simulink subsystem "leds"  (R2023b)
settings: Solver=VariableStepAuto  StartTime=0.0  StopTime=10.0  RelTol=1e-3
libraries: simulink x4, arduinolib x3
settings Model: Creator=Usuario_UMA  LastModifiedBy=fdcdm

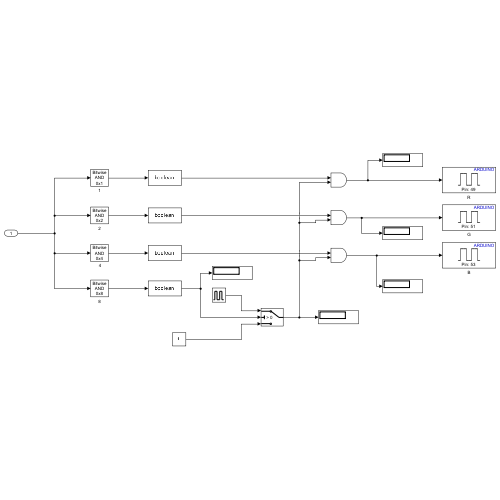
[thumbnail: Simulink's stored preview of the top-level diagram]
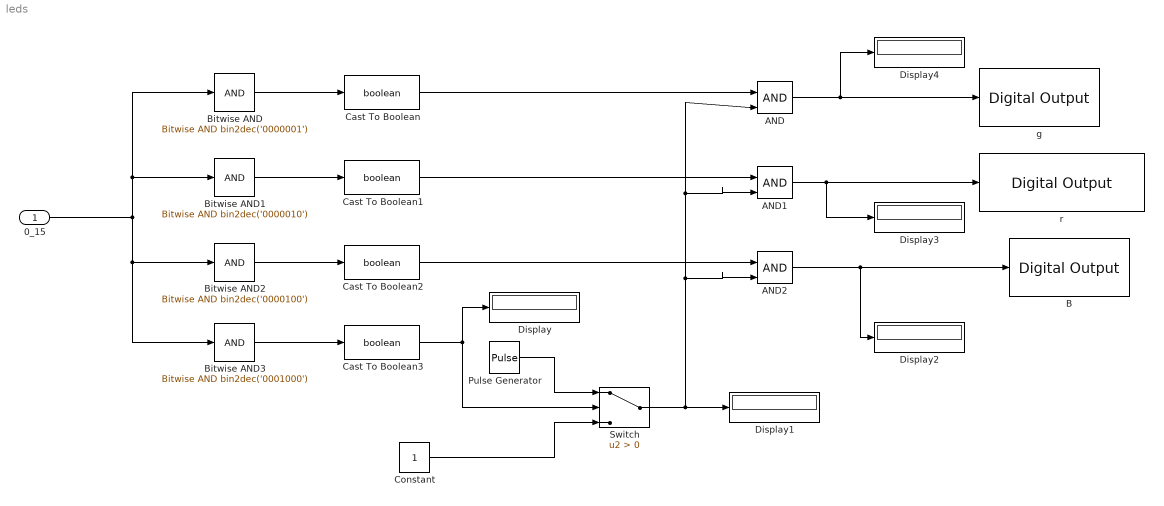
== system leds ==
  0_15 : Inport  OutDataTypeStr=uint8
  AND : Logic  IconShape=distinctive  AllPortsSameDT=off  OutDataTypeStr=boolean
  AND1 : Logic  IconShape=distinctive  AllPortsSameDT=off  OutDataTypeStr=boolean
  AND2 : Logic  IconShape=distinctive  AllPortsSameDT=off  OutDataTypeStr=boolean
  B : arduinolib/Digital Output  pinNumber=49  Direction=output  blockPlatform=arduino
  Bitwise AND : simulink/Logic and Bit Operations/Bitwise Operator  logicop=AND  UseBitMask=on  BitMask=bin2dec('0000001')  BitMaskRealWorld=Stored Integer
      settings: LibrarySourceBlock=|
      | simulink/Quick Insert/Logic and Bit
      | Operations/Bitwise AND
  Bitwise AND1 : simulink/Logic and Bit Operations/Bitwise Operator  logicop=AND  UseBitMask=on  BitMask=bin2dec('0000010')  BitMaskRealWorld=Stored Integer
      settings: LibrarySourceBlock=|
      | simulink/Quick Insert/Logic and Bit
      | Operations/Bitwise AND
  Bitwise AND2 : simulink/Logic and Bit Operations/Bitwise Operator  logicop=AND  UseBitMask=on  BitMask=bin2dec('0000100')  BitMaskRealWorld=Stored Integer
      settings: LibrarySourceBlock=|
      | simulink/Quick Insert/Logic and Bit
      | Operations/Bitwise AND
  Bitwise AND3 : simulink/Logic and Bit Operations/Bitwise Operator  logicop=AND  UseBitMask=on  BitMask=bin2dec('0001000')  BitMaskRealWorld=Stored Integer
      settings: LibrarySourceBlock=|
      | simulink/Quick Insert/Logic and Bit
      | Operations/Bitwise AND
  Cast To Boolean{,1..3} (4 alike) : DataTypeConversion  OutDataTypeStr=boolean  SaturateOnIntegerOverflow=off  RndMeth=Floor
  Constant : Constant
  Display{,1..4} (5 alike) : Display
  Pulse Generator : DiscretePulseGenerator  PulseType=Time based  Period=1  PulseWidth=50
  Switch : Switch  Criteria=u2 > Threshold  SaturateOnIntegerOverflow=off  InputSameDT=off
  g : arduinolib/Digital Output  pinNumber=51  Direction=output  blockPlatform=arduino
  r : arduinolib/Digital Output  pinNumber=53  Direction=output  blockPlatform=arduino
  wires:
  AND2/1 -> Display2/1, B/1
  AND1/1 -> Display3/1, r/1
  Switch/1 -> AND2/2, AND1/2, AND/2, Display1/1
  Pulse Generator/1 -> Switch/1
  Cast To Boolean/1 -> AND/1
  Bitwise AND3/1 -> Cast To Boolean3/1
  0_15/1 -> Bitwise AND/1, Bitwise AND1/1, Bitwise AND2/1, Bitwise AND3/1
  Constant/1 -> Switch/3
  Cast To Boolean1/1 -> AND1/1
  Bitwise AND/1 -> Cast To Boolean/1
  AND/1 -> Display4/1, g/1
  Cast To Boolean2/1 -> AND2/1
  Bitwise AND1/1 -> Cast To Boolean1/1
  Cast To Boolean3/1 -> Display/1, Switch/2
  Bitwise AND2/1 -> Cast To Boolean2/1
